simulink model "MPC_on_FCC"  (R2016a)
settings: Solver=ode45  StartTime=0.0  StopTime=20000  FixedStep=Ts  RelTol=1e-3
values from neighbouring files (symbols this model uses):
  P00 = [3 3 3 3; 3 3 3 3; 3 3 3 3; 3 3 3 3]    [filterParameters.m]
undefined symbols (not defined in the file or in its folder): X0, Yref
settings Model: Creator=hp  LastModifiedBy=hp
settings SolverCC: AutoInsertRateTranBlk=on
settings DataIOCC: SaveState=on  LoggingToFile=on

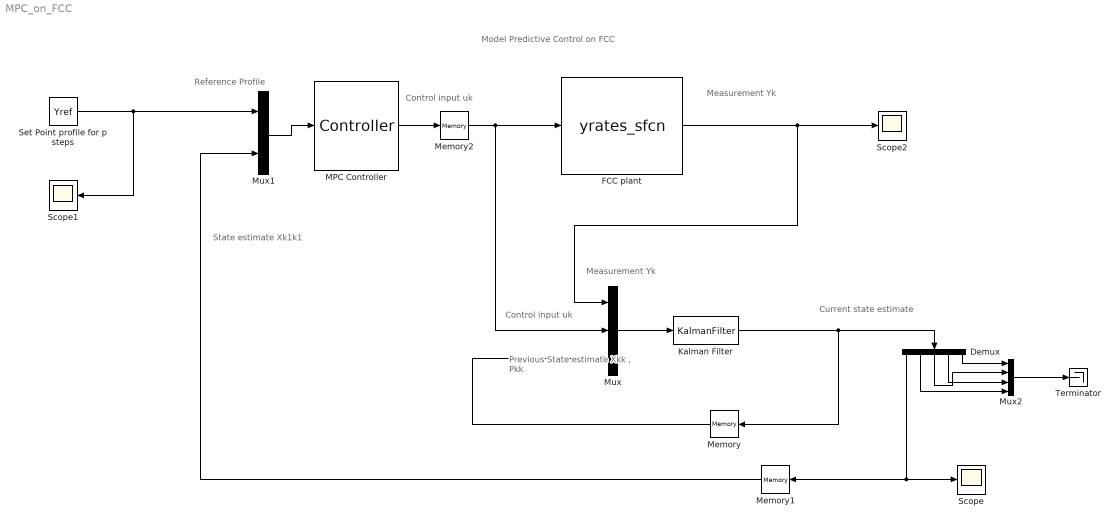
== system MPC_on_FCC ==
  note: Model Predictive Control on FCC
  note: Current state estimate
  note: Previous
      | State estimate Xkk , Pkk
  note: Control input uk
  note: Measurement Yk
  note: Control input uk
  note: Reference Profile
  note: State
      | estimate Xk1k1
  note: Measurement Yk
  Demux : Demux  Outputs=5
  FCC plant : S-Function  FunctionName=yrates_sfcn  Parameters=Y0  SFunctionDeploymentMode=off  EnableBusSupport=off
  Kalman Filter : MATLABFcn  MATLABFcn=KalmanFilter
  MPC Controller : MATLABFcn  MATLABFcn=Controller  Output1D=off
  Memory : Memory  X0=[X0; reshape(P00,[],1)]  InheritSampleTime=on  LinearizeAsDelay=on
  Memory1 : Memory  X0=X0  InheritSampleTime=on  LinearizeAsDelay=on
  Memory2 : Memory  X0=[0; 0]
  Mux : Mux  Inputs=3
  Mux1 : Mux  Inputs=2
  Mux2 : Mux
  Scope : Scope
  Scope1 : Scope
  Scope2 : Scope
  Set Point profile for p steps : Constant  Value=Yref  VectorParams1D=off
  Terminator : Terminator
  wires:
  Mux1/1 -> MPC Controller/1
  Mux/1 -> Kalman Filter/1
  Kalman Filter/1 -> Memory/1, Demux/1
  Memory/1 -> Mux/3
  Demux/1 -> Memory1/1, Scope/1
  FCC plant/1 -> Mux/1, Scope2/1
  Set Point profile for p steps/1 -> Scope1/1, Mux1/1
  Memory1/1 -> Mux1/2
  Mux2/1 -> Terminator/1
  MPC Controller/1 -> Memory2/1
  Memory2/1 -> Mux/2, FCC plant/1
  Demux/2 -> Mux2/4
  Demux/3 -> Mux2/2
  Demux/4 -> Mux2/3
  Demux/5 -> Mux2/1
